simulink model "additionneur_complet"  (R2024b)
settings: Solver=FixedStepDiscrete  StartTime=0.0  StopTime=10.0  RelTol=1e-3
libraries: hdlsllib x9
settings Model: DataTypeOverride=Off  Creator=User  LastModifiedBy=User
settings SolverCC: AlgebraicLoopSolver=TrustRegion
settings DataIOCC: LimitDataPoints=on  SaveOutput=off  SaveTime=off
settings OptimizationCC: BlockReduction=off  ConditionallyExecuteInputs=off  DefaultParameterBehavior=Inlined  LifeSpan=inf
settings DebuggingCC: AlgebraicLoopMsg=error  SingleTaskRateTransMsg=error  UnconnectedInputMsg=warning  UnconnectedOutputMsg=warning  UnconnectedLineMsg=warning  AllowSymbolicDim=off  StrictBusMsg=ErrorOnBusTreatedAsVector  SFUnexpectedBacktrackingDiag=warning  SFNoUnconditionalDefaultTransitionDiag=warning  SFExecutionAtInitializationDiag=none  ArithmeticOperatorsInVariantConditions=warning
settings HardwareCC: ProdBitPerPointer=32  ProdBitPerSizeT=32  ProdBitPerPtrDiffT=32  ProdLargestAtomicFloat=None  ProdIntDivRoundTo=Undefined  ProdEndianess=Unspecified  ProdWordSize=32  ProdHWDeviceType=ASIC/FPGA->ASIC/FPGA  ProdEqTarget=off
settings ModelReferenceCC: EnableRefExpFcnMdlSchedulingChecks=on
settings SFSimCC: SimUseLocalCustomCode=off  CustomCodeUndefinedFunction=UseInterfaceOnly
settings RTWCC: RTWUseLocalCustomCode=off  GPUComputeCapability=3.5
settings CodeAppCC: StateflowObjectComments=on
settings GRTTargetCC: TargetLangStandard=C89/C90 (ANSI)
settings ConfigComp: CovScope=ReferencedModels  CovMetricSettings=dw  CovSaveCumulativeToWorkspaceVar=on  CovSaveSingleToWorkspaceVar=on  CovExternalEMLEnable=off  CovSFcnEnable=off

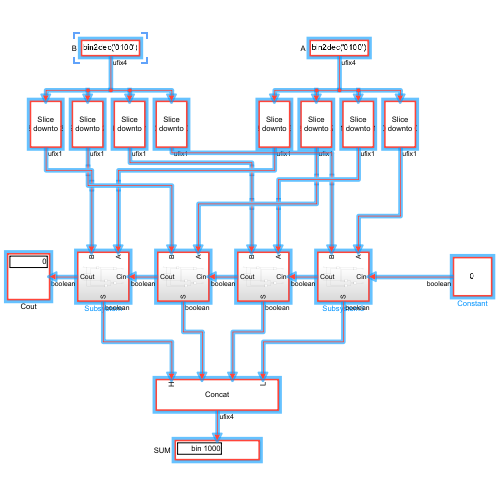
[thumbnail: Simulink's stored preview of the top-level diagram]
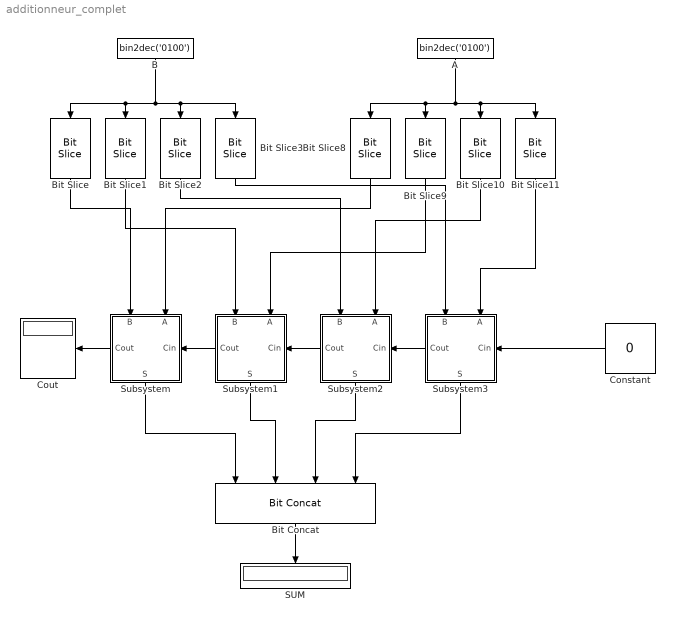
== system additionneur_complet ==
  A : Constant  Value=bin2dec('0100')  OutDataTypeStr=fixdt(0,4,0)  SampleTime=0
  B : Constant  Value=bin2dec('0100')  OutDataTypeStr=fixdt(0,4,0)  SampleTime=0
  Bit Concat : hdlsllib/Logic and Bit Operations/Bit Concat  numInputs=4
  Bit Slice : hdlsllib/Logic and Bit Operations/Bit Slice  lidx=3  ridx=3
  Bit Slice1 : hdlsllib/Logic and Bit Operations/Bit Slice  lidx=2  ridx=2
  Bit Slice10 : hdlsllib/Logic and Bit Operations/Bit Slice  lidx=1  ridx=1
  Bit Slice11 : hdlsllib/Logic and Bit Operations/Bit Slice  lidx=0  ridx=0
  Bit Slice2 : hdlsllib/Logic and Bit Operations/Bit Slice  lidx=1  ridx=1
  Bit Slice3 : hdlsllib/Logic and Bit Operations/Bit Slice  lidx=0  ridx=0
  Bit Slice8 : hdlsllib/Logic and Bit Operations/Bit Slice  lidx=3  ridx=3
  Bit Slice9 : hdlsllib/Logic and Bit Operations/Bit Slice  lidx=2  ridx=2
  Constant : Constant  Value=0  OutDataTypeStr=boolean  SampleTime=0
  Cout : Display
  SUM : Display
      settings: Format=binary (Stored Integer)
  Subsystem : Subsystem
      settings: PortSchema="{\"entries\":[{\"content\":{\"sides\":[{\"content\":{\"connectorIds\":[\"Out2\"]},\"type\":\"ConnectorPlacement.EquallySpacedRectSide\",\"uuid\":\"ce4c80a8-1d7e-4cb9-807c-e54a81683d65\"},{\"content\":{\"connectorIds\":[\"In3\"],\"side\":\"RIGHT\"},\"type\":\"ConnectorPlacement.EquallySpacedRectSide\",\"uuid\":\"22afab54-bb23-4c20-a70d-62308acc90fd\"},{\"content\":{\"connectorIds\":[\"In1\",\"In2\"],\"side\":\"TOP\"},\"type\":\"ConnectorPlacement.EquallySpacedRectSide\",\"uuid\":\"971c3cbb-79a1-4d7c-8fe4-4b61cf77d527\"},{\"content\":{\"connectorIds\":[\"Out1\"],\"side\":\"BOTTOM\"},\"type\":\"ConnectorPlacement.EquallySpacedRectSide\",\"uuid\":\"83a48bba-1c98-44ed-bf24-43217ef05ee8\"}]},\"type\":\"ConnectorPlacement.EquallySpacedConnector\",\"uuid\":\"226a0f1d-9266-4b5a-b9ed-ab63fef8e516\"}],\"packageUris\":[\"http://schema.mathworks.com/mf0/Connector/R2020b\"],\"version\":\"1.0\"}"
  Subsystem1 : Subsystem
      settings: PortSchema="{\"entries\":[{\"content\":{\"sides\":[{\"content\":{\"connectorIds\":[\"Out2\"]},\"type\":\"ConnectorPlacement.EquallySpacedRectSide\",\"uuid\":\"ce4c80a8-1d7e-4cb9-807c-e54a81683d65\"},{\"content\":{\"connectorIds\":[\"In3\"],\"side\":\"RIGHT\"},\"type\":\"ConnectorPlacement.EquallySpacedRectSide\",\"uuid\":\"22afab54-bb23-4c20-a70d-62308acc90fd\"},{\"content\":{\"connectorIds\":[\"In1\",\"In2\"],\"side\":\"TOP\"},\"type\":\"ConnectorPlacement.EquallySpacedRectSide\",\"uuid\":\"971c3cbb-79a1-4d7c-8fe4-4b61cf77d527\"},{\"content\":{\"connectorIds\":[\"Out1\"],\"side\":\"BOTTOM\"},\"type\":\"ConnectorPlacement.EquallySpacedRectSide\",\"uuid\":\"83a48bba-1c98-44ed-bf24-43217ef05ee8\"}]},\"type\":\"ConnectorPlacement.EquallySpacedConnector\",\"uuid\":\"226a0f1d-9266-4b5a-b9ed-ab63fef8e516\"}],\"packageUris\":[\"http://schema.mathworks.com/mf0/Connector/R2020b\"],\"version\":\"1.0\"}"
  Subsystem2 : Subsystem
      settings: PortSchema="{\"entries\":[{\"content\":{\"sides\":[{\"content\":{\"connectorIds\":[\"Out2\"]},\"type\":\"ConnectorPlacement.EquallySpacedRectSide\",\"uuid\":\"ce4c80a8-1d7e-4cb9-807c-e54a81683d65\"},{\"content\":{\"connectorIds\":[\"In3\"],\"side\":\"RIGHT\"},\"type\":\"ConnectorPlacement.EquallySpacedRectSide\",\"uuid\":\"22afab54-bb23-4c20-a70d-62308acc90fd\"},{\"content\":{\"connectorIds\":[\"In1\",\"In2\"],\"side\":\"TOP\"},\"type\":\"ConnectorPlacement.EquallySpacedRectSide\",\"uuid\":\"971c3cbb-79a1-4d7c-8fe4-4b61cf77d527\"},{\"content\":{\"connectorIds\":[\"Out1\"],\"side\":\"BOTTOM\"},\"type\":\"ConnectorPlacement.EquallySpacedRectSide\",\"uuid\":\"83a48bba-1c98-44ed-bf24-43217ef05ee8\"}]},\"type\":\"ConnectorPlacement.EquallySpacedConnector\",\"uuid\":\"226a0f1d-9266-4b5a-b9ed-ab63fef8e516\"}],\"packageUris\":[\"http://schema.mathworks.com/mf0/Connector/R2020b\"],\"version\":\"1.0\"}"
  Subsystem3 : Subsystem
      settings: PortSchema="{\"entries\":[{\"content\":{\"sides\":[{\"content\":{\"connectorIds\":[\"Out2\"]},\"type\":\"ConnectorPlacement.EquallySpacedRectSide\",\"uuid\":\"ce4c80a8-1d7e-4cb9-807c-e54a81683d65\"},{\"content\":{\"connectorIds\":[\"In3\"],\"side\":\"RIGHT\"},\"type\":\"ConnectorPlacement.EquallySpacedRectSide\",\"uuid\":\"22afab54-bb23-4c20-a70d-62308acc90fd\"},{\"content\":{\"connectorIds\":[\"In1\",\"In2\"],\"side\":\"TOP\"},\"type\":\"ConnectorPlacement.EquallySpacedRectSide\",\"uuid\":\"971c3cbb-79a1-4d7c-8fe4-4b61cf77d527\"},{\"content\":{\"connectorIds\":[\"Out1\"],\"side\":\"BOTTOM\"},\"type\":\"ConnectorPlacement.EquallySpacedRectSide\",\"uuid\":\"83a48bba-1c98-44ed-bf24-43217ef05ee8\"}]},\"type\":\"ConnectorPlacement.EquallySpacedConnector\",\"uuid\":\"226a0f1d-9266-4b5a-b9ed-ab63fef8e516\"}],\"packageUris\":[\"http://schema.mathworks.com/mf0/Connector/R2020b\"],\"version\":\"1.0\"}"
  wires:
  Subsystem1/2(Cout) -> Subsystem/3(Cin)
  Subsystem2/2(Cout) -> Subsystem1/3(Cin)
  Subsystem3/2(Cout) -> Subsystem2/3(Cin)
  Subsystem/1(S) -> Bit Concat/1
  Subsystem1/1(S) -> Bit Concat/2
  Subsystem2/1(S) -> Bit Concat/3
  Subsystem3/1(S) -> Bit Concat/4
  Bit Concat/1 -> SUM/1
  B/1 -> Bit Slice2/1, Bit Slice3/1, Bit Slice1/1, Bit Slice/1
  A/1 -> Bit Slice10/1, Bit Slice11/1, Bit Slice9/1, Bit Slice8/1
  Subsystem/2(Cout) -> Cout/1
  Constant/1 -> Subsystem3/3(Cin)
  Bit Slice11/1 -> Subsystem3/2(A)
  Bit Slice10/1 -> Subsystem2/2(A)
  Bit Slice9/1 -> Subsystem1/2(A)
  Bit Slice8/1 -> Subsystem/2(A)
  Bit Slice/1 -> Subsystem/1(B)
  Bit Slice1/1 -> Subsystem1/1(B)
  Bit Slice2/1 -> Subsystem2/1(B)
  Bit Slice3/1 -> Subsystem3/1(B)

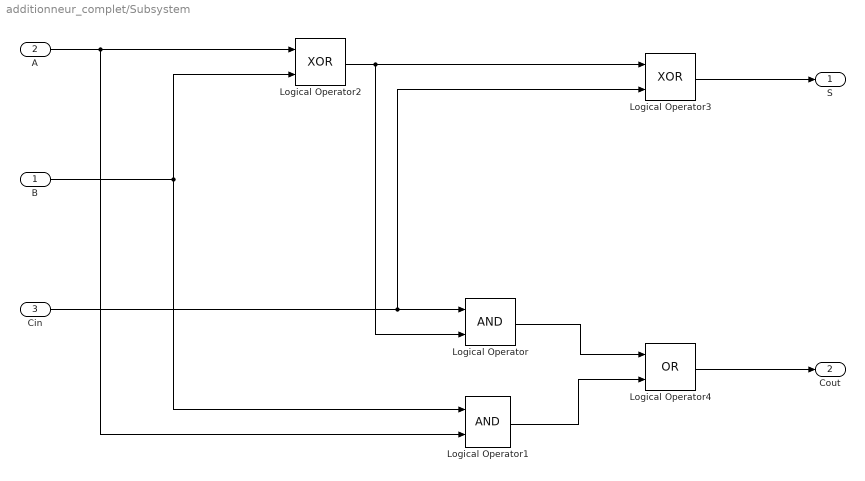
== system additionneur_complet/Subsystem ==
  B : Inport
  A : Inport  Port=2
  Cin : Inport  Port=3
  Logical Operator : Logic  AllPortsSameDT=off  OutDataTypeStr=boolean
  Logical Operator1 : Logic  AllPortsSameDT=off  OutDataTypeStr=boolean
  Logical Operator2 : Logic  Operator=XOR  AllPortsSameDT=off  OutDataTypeStr=boolean
  Logical Operator3 : Logic  Operator=XOR  AllPortsSameDT=off  OutDataTypeStr=boolean
  Logical Operator4 : Logic  Operator=OR  AllPortsSameDT=off  OutDataTypeStr=boolean
  S : Outport
  Cout : Outport  Port=2
  wires:
  A/1 -> Logical Operator1/2, Logical Operator2/1
  Logical Operator/1 -> Logical Operator4/1
  B/1 -> Logical Operator1/1, Logical Operator2/2
  Logical Operator3/1 -> S/1
  Logical Operator2/1 -> Logical Operator/2, Logical Operator3/1
  Cin/1 -> Logical Operator3/2, Logical Operator/1
  Logical Operator1/1 -> Logical Operator4/2
  Logical Operator4/1 -> Cout/1

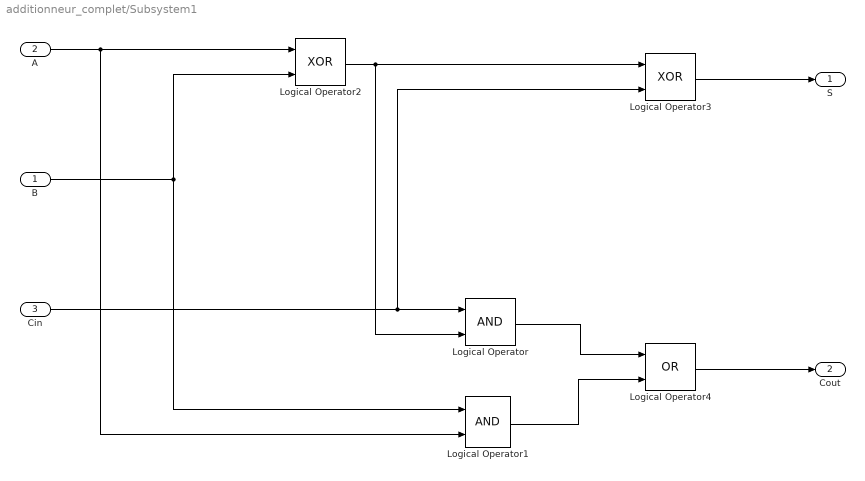
== system additionneur_complet/Subsystem1 ==
  B : Inport
  A : Inport  Port=2
  Cin : Inport  Port=3
  Logical Operator : Logic  AllPortsSameDT=off  OutDataTypeStr=boolean
  Logical Operator1 : Logic  AllPortsSameDT=off  OutDataTypeStr=boolean
  Logical Operator2 : Logic  Operator=XOR  AllPortsSameDT=off  OutDataTypeStr=boolean
  Logical Operator3 : Logic  Operator=XOR  AllPortsSameDT=off  OutDataTypeStr=boolean
  Logical Operator4 : Logic  Operator=OR  AllPortsSameDT=off  OutDataTypeStr=boolean
  S : Outport
  Cout : Outport  Port=2
  wires:
  A/1 -> Logical Operator1/2, Logical Operator2/1
  Logical Operator/1 -> Logical Operator4/1
  B/1 -> Logical Operator1/1, Logical Operator2/2
  Logical Operator3/1 -> S/1
  Logical Operator2/1 -> Logical Operator/2, Logical Operator3/1
  Cin/1 -> Logical Operator3/2, Logical Operator/1
  Logical Operator1/1 -> Logical Operator4/2
  Logical Operator4/1 -> Cout/1

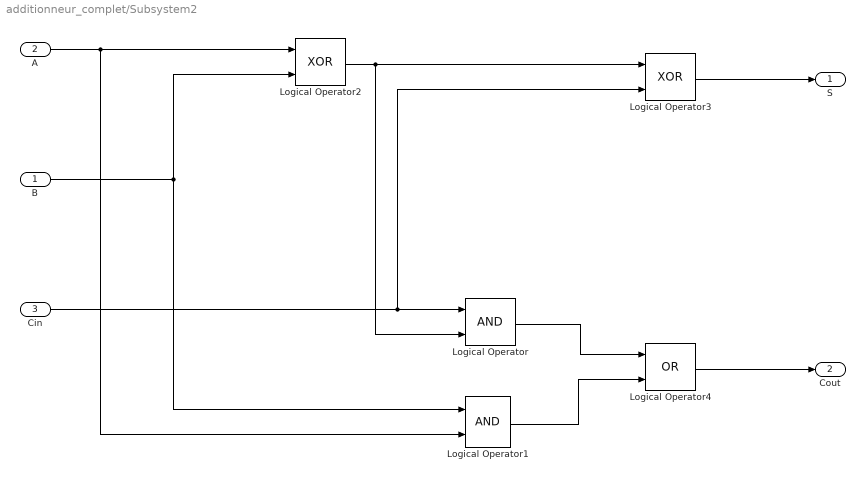
== system additionneur_complet/Subsystem2 ==
  B : Inport
  A : Inport  Port=2
  Cin : Inport  Port=3
  Logical Operator : Logic  AllPortsSameDT=off  OutDataTypeStr=boolean
  Logical Operator1 : Logic  AllPortsSameDT=off  OutDataTypeStr=boolean
  Logical Operator2 : Logic  Operator=XOR  AllPortsSameDT=off  OutDataTypeStr=boolean
  Logical Operator3 : Logic  Operator=XOR  AllPortsSameDT=off  OutDataTypeStr=boolean
  Logical Operator4 : Logic  Operator=OR  AllPortsSameDT=off  OutDataTypeStr=boolean
  S : Outport
  Cout : Outport  Port=2
  wires:
  A/1 -> Logical Operator1/2, Logical Operator2/1
  Logical Operator/1 -> Logical Operator4/1
  B/1 -> Logical Operator1/1, Logical Operator2/2
  Logical Operator3/1 -> S/1
  Logical Operator2/1 -> Logical Operator/2, Logical Operator3/1
  Cin/1 -> Logical Operator3/2, Logical Operator/1
  Logical Operator1/1 -> Logical Operator4/2
  Logical Operator4/1 -> Cout/1

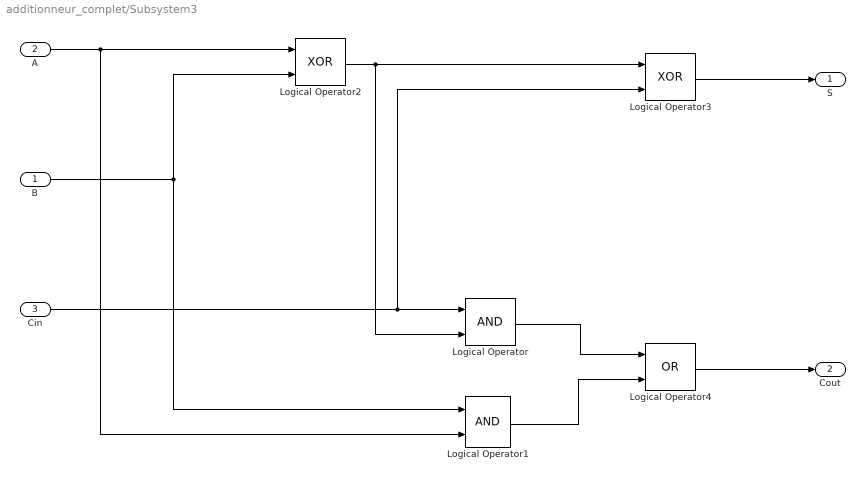
== system additionneur_complet/Subsystem3 ==
  B : Inport
  A : Inport  Port=2
  Cin : Inport  Port=3
  Logical Operator : Logic  AllPortsSameDT=off  OutDataTypeStr=boolean
  Logical Operator1 : Logic  AllPortsSameDT=off  OutDataTypeStr=boolean
  Logical Operator2 : Logic  Operator=XOR  AllPortsSameDT=off  OutDataTypeStr=boolean
  Logical Operator3 : Logic  Operator=XOR  AllPortsSameDT=off  OutDataTypeStr=boolean
  Logical Operator4 : Logic  Operator=OR  AllPortsSameDT=off  OutDataTypeStr=boolean
  S : Outport
  Cout : Outport  Port=2
  wires:
  A/1 -> Logical Operator1/2, Logical Operator2/1
  Logical Operator/1 -> Logical Operator4/1
  B/1 -> Logical Operator1/1, Logical Operator2/2
  Logical Operator3/1 -> S/1
  Logical Operator2/1 -> Logical Operator/2, Logical Operator3/1
  Cin/1 -> Logical Operator3/2, Logical Operator/1
  Logical Operator1/1 -> Logical Operator4/2
  Logical Operator4/1 -> Cout/1
